simulink model "SIR_model"  (R2020a)
settings: Solver=VariableStepAuto  StartTime=0.0  StopTime=tf  RelTol=1e-3
undefined symbols (not defined in the file): beta, gamma, mu, x0
settings Model: OrderedModelArguments=off  Creator=ciro  LastModifiedBy=ciro

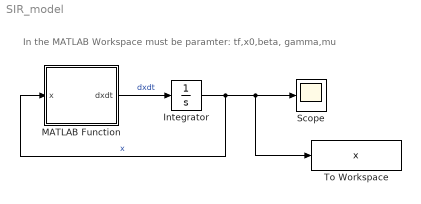
== system SIR_model ==
  note: In the MATLAB Workspace must be paramter: tf,x0,beta, gamma,mu
  Integrator : Integrator  InitialCondition=x0
  MATLAB Function : MATLAB Function  TreatAsAtomicUnit=on
  Scope : Scope
  To Workspace : ToWorkspace  VariableName=x  SaveFormat=Timeseries  SampleTime=-1
  wires:
  MATLAB Function/1(dxdt) -> Integrator/1  "dxdt"
  Integrator/1 -> To Workspace/1, Scope/1, MATLAB Function/1(x)  "x"

== matlab function SIR_model/MATLAB Function ==
  data: x input; dxdt output; mu parameter; gamma parameter; beta parameter
function dxdt  = SIR(x, mu, gamma, beta)
    dxdt = zeros(size(x));
    dxdt(1) = mu - mu*x(1) - beta*x(1)*x(2);
    dxdt(2) = beta*x(1)*x(2) - (gamma + mu)*x(2);
end
